simulink model "seti_ct"  (Simulink 6.2)
settings: Solver=ode45  StartTime=0.0  StopTime=100000  RelTol=1e-3
values from neighbouring files (symbols this model uses):
  bigColBits = 0    [address_gen_dram_mask.m]
  bigRowBits = log2(bigRowLength)    [address_gen_dram_mask.m]
  smallColBits = 0    [address_gen_dram_mask.m]
  smallRowBits = log2(smallRowLength)    [address_gen_dram_mask.m]
libraries: xbsIndex_r3 x487, xps_library x45, casper_library x18, fft_library x1
(part 1 of 3)
settings Model: LastModifiedBy=lspitler
settings DebuggingCC: SolverPrmCheckMsg=warning

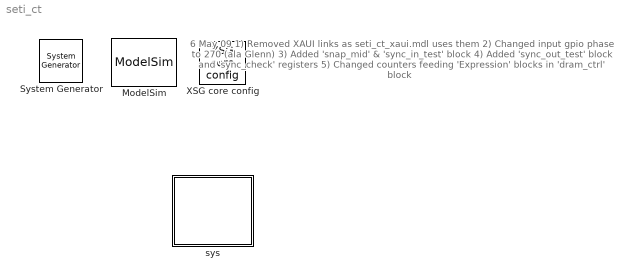
== system seti_ct ==
  note: 6 May 09
      | 1) Removed XAUI links as seti_ct_xaui.mdl uses them
      | 2) Changed input gpio phase to 270 (ala Glenn)
      | 3) Added 'snap_mid' & 'sync_in_test' block
      | 4) Added 'sync_out_test' block and 'sync_check' registers
      | 5) Changed counters feeding 'Expression' blocks
      | in 'dram_ctrl' block
  " System Generator" : xbsIndex_r3/ System Generator  Tag=genX  xilinxfamily=Virtex2P  part=xc2vp70  speed=-7  package=ff1704  synthesis_tool=XST  directory=./seti_ct/sysgen  testbench=off  simulink_period=1  sysclk_period=4.878  incr_netlist=off  trim_vbits=Everywhere in SubSystem  dbl_ovrd=According to Block Masks  core_generation=According to Block Masks  run_coregen=off  deprecated_control=off  eval_field=0
      settings: AttributesFormatString=System\nGenerator
  ModelSim : xbsIndex_r3/ModelSim  dir=./modelsim  waveform=on  leave_open=on  skip_compile=off  custom_scripts=on  post_vsim_script=dram_sim.do  startup_timeout=3600
  XSG core config : xps_library/XSG core config  Tag=xps:xsg  hw_sys=BEE2_usr  ibob_linux=off  clk_src=usr_clk2x  gpio_clk_io_group=iBOB:sma  gpio_clk_bit_index=0  clk_rate=205  sample_period=1  synthesis_tool=XST  mpc_type=powerpc405
  sys : Subsystem  mask{numSpecs=2^15, length=2^12, ct_delay=50}
      mask prompts: numSpecs "Number of Specs?"; length "Length of Specs?"; ct_delay "CornerTurn Delay"

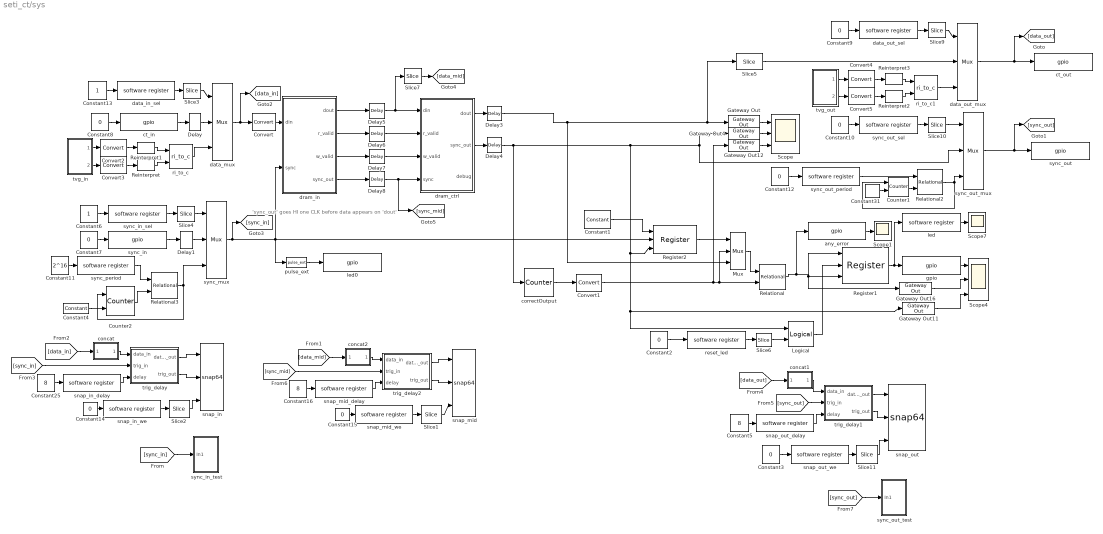
== system seti_ct/sys ==
  note: 'sync_out' goes HI
      | one CLK before
      | data appears on 'dout'
  Constant1 : xbsIndex_r3/Constant  const=1  equ=P=C  arith_type=Unsigned  n_bits=1  bin_pt=0  opselect=C  inp2=PCIN>>17  opr=+  inp1=P  carry=CIN  iostate=0  explicit_period=on  period=1  dbl_ovrd=off
  Constant{2..3,7..10,12,14..15} (9 alike) : Constant  Value=0
  Constant11 : Constant  Value=2^16
  Constant13 : Constant
  Constant16 : Constant  Value=8
  Constant25 : Constant  Value=8
  Constant31 : xbsIndex_r3/Constant  const=1  equ=P=C  arith_type=Unsigned  n_bits=32  bin_pt=0  opselect=C  inp2=PCIN>>17  opr=+  inp1=P  carry=CIN  iostate=0  explicit_period=on  period=1  dbl_ovrd=off
  Constant4 : xbsIndex_r3/Constant  const=1  equ=P=C  arith_type=Unsigned  n_bits=32  bin_pt=0  opselect=C  inp2=PCIN>>17  opr=+  inp1=P  carry=CIN  iostate=0  explicit_period=on  period=1  dbl_ovrd=off
  Constant5 : Constant  Value=8
  Constant6 : Constant
  Convert : xbsIndex_r3/Convert  arith_type=Unsigned  n_bits=72  bin_pt=0  quantization=Truncate  overflow=Wrap  latency=0  explicit_period=off  period=1  dbl_ovrd=off  show_param=off  inserted_by_tool=off  pipeline=off
      settings: xl_area=[0, 0, 0, 0, 0, 0, 0]
  Convert1 : xbsIndex_r3/Convert  arith_type=Unsigned  n_bits=72  bin_pt=0  quantization=Truncate  overflow=Wrap  latency=0  explicit_period=off  period=1  dbl_ovrd=off  show_param=off  inserted_by_tool=off  pipeline=off
      settings: xl_area=[0, 0, 0, 0, 0, 0, 0]
  Convert{2..5} (4 alike) : xbsIndex_r3/Convert  arith_type=Unsigned  n_bits=18  bin_pt=0  quantization=Truncate  overflow=Wrap  latency=0  explicit_period=on  period=1  dbl_ovrd=off  show_param=off  inserted_by_tool=off  pipeline=off
      settings: xl_area=[0, 0, 0, 0, 0, 0, 0]
  Counter1 : xbsIndex_r3/Counter  cnt_type=Free Running  n_bits=32  bin_pt=0  arith_type=Unsigned  start_count=0  cnt_to=Inf  cnt_by_val=1  operation=Up  explicit_period=on  period=1  load_pin=on  rst=off  en=off  dbl_ovrd=off  show_param=off  use_rpm=on  gen_core=off
      settings: xl_area=[0, 0, 0, 0, 0, 0, 0]
  Counter2 : xbsIndex_r3/Counter  cnt_type=Free Running  n_bits=32  bin_pt=0  arith_type=Unsigned  start_count=0  cnt_to=Inf  cnt_by_val=1  operation=Up  explicit_period=on  period=1  load_pin=on  rst=off  en=off  dbl_ovrd=off  show_param=off  use_rpm=on  gen_core=off
      settings: xl_area=[0, 0, 0, 0, 0, 0, 0]
  Delay{,1,3..8} (8 alike) : xbsIndex_r3/Delay  latency=1  reg_retiming=off  explicit_period=off  period=1  en=off  accept_only_valid=off  init_zero=on  dbl_ovrd=off  show_param=off
      settings: xl_area=[0, 0, 0, 0, 0, 0, 0]
  Gateway Out{,4,11..12,16} (5 alike) : xbsIndex_r3/Gateway Out  output_type=Double  nbits=8  bin_pt=6  arith_type=Boolean  quantization=Truncate  overflow=Wrap  hdl_port=off  timing_constraint=None  locs_specified=off  LOCs={}  needs_fixed_name=off  show_param=off
      settings: xl_area=[0, 0, 0, 0, 0, 0, 0]
  Logical : xbsIndex_r3/Logical  logical_function=AND  inputs=2  precision=Full  arith_type=Unsigned  n_bits=8  bin_pt=2  align_bp=on  latency=0  explicit_period=off  period=1  en=off  dbl_ovrd=off  show_param=off
      settings: xl_area=[0, 0, 0, 0, 0, 0, 0]
  Mux : xbsIndex_r3/Mux  inputs=2  precision=Full  arith_type="Signed  (2's comp)"  n_bits=8  bin_pt=2  quantization=Truncate  overflow=Wrap  latency=0  explicit_period=off  period=1  en=off  dbl_ovrd=off  show_param=off  mux_type=off  use_rpm=off  gen_core=off
      settings: xl_area=[0, 0, 0, 0, 0, 0, 0]
  Register1 : xbsIndex_r3/Register  init=0  reg_only_valid=off  explicit_period=off  period=1  rst=on  en=on  out_en=off  dbl_ovrd=off  show_param=off
      settings: xl_area=[0, 0, 0, 0, 0, 0, 0]
  Register2 : xbsIndex_r3/Register  init=0  reg_only_valid=off  explicit_period=off  period=1  rst=on  en=on  out_en=off  dbl_ovrd=off  show_param=off
      settings: xl_area=[0, 0, 0, 0, 0, 0, 0]
  Reinterpret{,1..3} (4 alike) : xbsIndex_r3/Reinterpret  force_arith_type=on  arith_type="Signed  (2's comp)"  force_bin_pt=on  bin_pt=17  force_valid=on
  Relational : xbsIndex_r3/Relational  mode=a!=b  latency=1  explicit_period=off  period=1  en=off  dbl_ovrd=off  show_param=off
      settings: xl_area=[0, 0, 0, 0, 0, 0, 0]
  Relational2 : xbsIndex_r3/Relational  mode=a=b  latency=1  explicit_period=off  period=1  en=off  dbl_ovrd=off  show_param=off
      settings: xl_area=[0, 0, 0, 0, 0, 0, 0]
  Relational3 : xbsIndex_r3/Relational  mode=a=b  latency=1  explicit_period=on  period=1  en=off  dbl_ovrd=off  show_param=off
      settings: xl_area=[0, 0, 0, 0, 0, 0, 0]
  Scope : Scope  NumInputPorts=3
      settings: YMin=-1~-1~0  YMax=1~1~1750  SaveName=ScopeData9
  Scope1 : Scope
      settings: SaveName=ScopeData12
  Scope4 : Scope  NumInputPorts=3
      settings: YMin=-1~-1~-1  YMax=1~1~1  SaveName=ScopeData10
  Scope7 : Scope
      settings: SaveName=ScopeData13
  Slice{1..2,6,11} (4 alike) : xbsIndex_r3/Slice  mode=Lower Bit Location + Width  nbits=1  bit1=0  base1=MSB of Input  bit0=0  base0=LSB of Input  boolean_output=on  explicit_period=off  period=1  dbl_ovrd=off
  Slice{3..4,9..10} (4 alike) : xbsIndex_r3/Slice  mode=Lower Bit Location + Width  nbits=1  bit1=0  base1=MSB of Input  bit0=0  base0=LSB of Input  boolean_output=off  explicit_period=off  period=1  dbl_ovrd=off
  Slice5 : xbsIndex_r3/Slice  mode=Lower Bit Location + Width  nbits=36  bit1=0  base1=MSB of Input  bit0=0  base0=LSB of Input  boolean_output=off  explicit_period=off  period=1  dbl_ovrd=off
  Slice7 : xbsIndex_r3/Slice  mode=Lower Bit Location + Width  nbits=36  bit1=0  base1=MSB of Input  bit0=0  base0=LSB of Input  boolean_output=off  explicit_period=off  period=1  dbl_ovrd=off
  any_error : xps_library/gpio  Tag=xps:gpio  io_group=BEE2_usr:led  io_dir=out  arith_type=Unsigned  bitwidth=1  bin_pt=0  bit_index=4  sample_period=1  use_single_ended=off  use_ddr=off  reg_iob=off  reg_clk_phase=0  termination=None
  concat : Subsystem
  concat1 : Subsystem
  concat2 : Subsystem
  correctOutput : xbsIndex_r3/Counter  cnt_type=Free Running  n_bits=log2(length)+log2(numSpecs)  bin_pt=0  arith_type=Unsigned  start_count=0  cnt_to=Inf  cnt_by_val=1  operation=Up  explicit_period=off  period=1  load_pin=off  rst=on  en=off  dbl_ovrd=off  show_param=off  use_rpm=on  gen_core=off
      settings: xl_area=[0, 0, 0, 0, 0, 0, 0]
  ct_in : xps_library/gpio  Tag=xps:gpio  io_group=BEE2_usr:rightlink  io_dir=in  arith_type=Unsigned  bitwidth=36  bin_pt=0  bit_index=[0:35]  sample_period=1  use_single_ended=off  use_ddr=off  reg_iob=on  reg_clk_phase=270  termination=None
  ct_out : xps_library/gpio  Tag=xps:gpio  io_group=BEE2_usr:leftlink  io_dir=out  arith_type=Unsigned  bitwidth=36  bin_pt=0  bit_index=[0:35]  sample_period=1  use_single_ended=off  use_ddr=off  reg_iob=on  reg_clk_phase=0  termination=None
  data_in_sel : xps_library/software register  Tag=xps:sw_reg  io_dir=From Processor  arith_type=Unsigned  bitwidth=32  bin_pt=0  sample_period=1  gw_name=seti_ct_sys_data_in_sel_user_data_out
  data_mux : xbsIndex_r3/Mux  inputs=2  precision=Full  arith_type="Signed  (2's comp)"  n_bits=8  bin_pt=2  quantization=Truncate  overflow=Wrap  latency=2  explicit_period=on  period=1  en=off  dbl_ovrd=off  show_param=off  mux_type=off  use_rpm=off  gen_core=off
      settings: xl_area=[0, 0, 0, 0, 0, 0, 0]
  data_out_mux : xbsIndex_r3/Mux  inputs=2  precision=Full  arith_type="Signed  (2's comp)"  n_bits=8  bin_pt=2  quantization=Truncate  overflow=Wrap  latency=2  explicit_period=on  period=1  en=off  dbl_ovrd=off  show_param=off  mux_type=off  use_rpm=off  gen_core=off
      settings: xl_area=[0, 0, 0, 0, 0, 0, 0]
  data_out_sel : xps_library/software register  Tag=xps:sw_reg  io_dir=From Processor  arith_type=Unsigned  bitwidth=32  bin_pt=0  sample_period=1  gw_name=seti_ct_sys_data_out_sel_user_data_out
  dram_ctrl : Subsystem  mask{spec_len=log2(length), num_spec=log2(numSpecs), ct_delay=ct_delay}
      mask prompts: spec_len "Spectrum Length (2^?)"; num_spec "Number of Spectra (2^?)"; ct_delay "Counterturn Delay"
  dram_in : Subsystem  mask{spec_len=log2(length)}
      mask prompts: spec_len "Spectrum Length (2^?)"
  gpio : xps_library/gpio  Tag=xps:gpio  io_group=BEE2_usr:led  io_dir=out  arith_type=Unsigned  bitwidth=1  bin_pt=0  bit_index=5  sample_period=1  use_single_ended=off  use_ddr=off  reg_iob=off  reg_clk_phase=0  termination=None
  led : xps_library/software register  Tag=xps:sw_reg  io_dir=To Processor  arith_type=Unsigned  bitwidth=32  bin_pt=0  sample_period=1  gw_name=seti_ct_sys_led_user_data_in
  led0 : xps_library/gpio  Tag=xps:gpio  io_group=BEE2_usr:led  io_dir=out  arith_type=Boolean  bitwidth=1  bin_pt=0  bit_index=0  sample_period=1  use_single_ended=off  use_ddr=off  reg_iob=on  reg_clk_phase=0  termination=None
  pulse_ext : casper_library/Misc/pulse_ext  pulse_len=2^25
  reset_led : xps_library/software register  Tag=xps:sw_reg  io_dir=From Processor  arith_type=Unsigned  bitwidth=32  bin_pt=0  sample_period=1  gw_name=seti_ct_sys_reset_led_user_data_out
  ri_to_c : casper_library/Misc/ri_to_c
  ri_to_c1 : casper_library/Misc/ri_to_c
  snap_in : casper_library/Scopes/snap64  nsamples=12
  snap_in_delay : xps_library/software register  Tag=xps:sw_reg  io_dir=From Processor  arith_type=Unsigned  bitwidth=32  bin_pt=0  sample_period=1  gw_name=seti_ct_sys_snap_in_delay_user_data_out
  snap_in_we : xps_library/software register  Tag=xps:sw_reg  io_dir=From Processor  arith_type=Unsigned  bitwidth=32  bin_pt=0  sample_period=1  gw_name=seti_ct_sys_snap_in_we_user_data_out
  snap_mid : casper_library/Scopes/snap64  nsamples=12
  snap_mid_delay : xps_library/software register  Tag=xps:sw_reg  io_dir=From Processor  arith_type=Unsigned  bitwidth=32  bin_pt=0  sample_period=1  gw_name=seti_ct_sys_snap_mid_delay_user_data_out
  snap_mid_we : xps_library/software register  Tag=xps:sw_reg  io_dir=From Processor  arith_type=Unsigned  bitwidth=32  bin_pt=0  sample_period=1  gw_name=seti_ct_sys_snap_mid_we_user_data_out
  snap_out : casper_library/Scopes/snap64  nsamples=11
  snap_out_delay : xps_library/software register  Tag=xps:sw_reg  io_dir=From Processor  arith_type=Unsigned  bitwidth=32  bin_pt=0  sample_period=1  gw_name=seti_ct_sys_snap_out_delay_user_data_out
  snap_out_we : xps_library/software register  Tag=xps:sw_reg  io_dir=From Processor  arith_type=Unsigned  bitwidth=32  bin_pt=0  sample_period=1  gw_name=seti_ct_sys_snap_out_we_user_data_out
  sync_in : xps_library/gpio  Tag=xps:gpio  io_group=BEE2_usr:rightlink  io_dir=in  arith_type=Boolean  bitwidth=1  bin_pt=0  bit_index=36  sample_period=1  use_single_ended=off  use_ddr=off  reg_iob=on  reg_clk_phase=270  termination=None
  sync_in_sel : xps_library/software register  Tag=xps:sw_reg  io_dir=From Processor  arith_type=Unsigned  bitwidth=32  bin_pt=0  sample_period=1  gw_name=seti_ct_sys_sync_in_sel_user_data_out
  sync_in_test : Subsystem
  sync_mux : xbsIndex_r3/Mux  inputs=2  precision=Full  arith_type="Signed  (2's comp)"  n_bits=8  bin_pt=2  quantization=Truncate  overflow=Wrap  latency=2  explicit_period=on  period=1  en=off  dbl_ovrd=off  show_param=off  mux_type=off  use_rpm=off  gen_core=off
      settings: xl_area=[0, 0, 0, 0, 0, 0, 0]
  sync_out : xps_library/gpio  Tag=xps:gpio  io_group=BEE2_usr:leftlink  io_dir=out  arith_type=Boolean  bitwidth=1  bin_pt=0  bit_index=36  sample_period=1  use_single_ended=off  use_ddr=off  reg_iob=on  reg_clk_phase=0  termination=None
  sync_out_mux : xbsIndex_r3/Mux  inputs=2  precision=Full  arith_type="Signed  (2's comp)"  n_bits=8  bin_pt=2  quantization=Truncate  overflow=Wrap  latency=2  explicit_period=on  period=1  en=off  dbl_ovrd=off  show_param=off  mux_type=off  use_rpm=off  gen_core=off
      settings: xl_area=[0, 0, 0, 0, 0, 0, 0]
  sync_out_period : xps_library/software register  Tag=xps:sw_reg  io_dir=From Processor  arith_type=Unsigned  bitwidth=32  bin_pt=0  sample_period=1  gw_name=seti_ct_sys_sync_out_period_user_data_out
  sync_out_sel : xps_library/software register  Tag=xps:sw_reg  io_dir=From Processor  arith_type=Unsigned  bitwidth=32  bin_pt=0  sample_period=1  gw_name=seti_ct_sys_sync_out_sel_user_data_out
  sync_out_test : Subsystem
  sync_period : xps_library/software register  Tag=xps:sw_reg  io_dir=From Processor  arith_type=Unsigned  bitwidth=32  bin_pt=0  sample_period=1  gw_name=seti_ct_sys_sync_period_user_data_out
  trig_delay : Subsystem
  trig_delay1 : Subsystem
  trig_delay2 : Subsystem
  tvg_in : Subsystem
  tvg_out : Subsystem
  wires:
  dram_in/2(r_valid) -> Delay6/1
  dram_in/3(w_valid) -> Delay7/1
  dram_in/4(sync_out) -> Delay8/1
  dram_in/1(dout) -> Delay5/1
  Convert/1 -> dram_in/1(din)
  dram_ctrl/1(dout) -> Delay3/1
  dram_ctrl/2(sync_out) -> Delay4/1
  Gateway Out/1 -> Scope/1
  correctOutput/1 -> Convert1/1
  Relational/1 -> Register1/3, Register1/1, Gateway Out16/1, any_error/1
  Register1/1 -> gpio/1, led/1
  gpio/1 -> Scope4/1
  Mux/1 -> Relational/1
  Register2/1 -> Mux/1
  Constant1/1 -> Register2/1
  Gateway Out12/1 -> Scope/3
  Gateway Out16/1 -> Scope4/2
  Gateway Out11/1 -> Scope4/3
  led/1 -> Scope7/1
  reset_led/1 -> Slice6/1
  Constant2/1 -> reset_led/1
  Slice6/1 -> Logical/2
  Logical/1 -> Register1/2
  any_error/1 -> Scope1/1
  Convert1/1 -> Relational/2, Mux/2, Gateway Out12/1
  data_in_sel/1 -> Slice3/1
  Constant13/1 -> data_in_sel/1
  Slice3/1 -> data_mux/1
  ri_to_c/1 -> data_mux/3
  ct_in/1 -> Delay/1
  sync_in_sel/1 -> Slice4/1
  Constant6/1 -> sync_in_sel/1
  Slice4/1 -> sync_mux/1
  sync_in/1 -> Delay1/1
  Constant7/1 -> sync_in/1
  sync_mux/1 -> Register2/2, dram_in/2(sync), pulse_ext/1, [sync_in]
  Constant8/1 -> ct_in/1
  Gateway Out4/1 -> Scope/2
  Convert2/1 -> Reinterpret1/1
  Convert3/1 -> Reinterpret/1
  tvg_in/1(re_out) -> Convert2/1
  tvg_in/2(im_out) -> Convert3/1
  Reinterpret1/1 -> ri_to_c/1
  Reinterpret/1 -> ri_to_c/2
  data_out_sel/1 -> Slice9/1
  Constant9/1 -> data_out_sel/1
  Slice9/1 -> data_out_mux/1
  ri_to_c1/1 -> data_out_mux/3
  Slice5/1 -> data_out_mux/2
  data_out_mux/1 -> [data_out], ct_out/1
  Convert4/1 -> Reinterpret3/1
  Convert5/1 -> Reinterpret2/1
  tvg_out/1(re_out) -> Convert4/1
  tvg_out/2(im_out) -> Convert5/1
  Reinterpret3/1 -> ri_to_c1/1
  Reinterpret2/1 -> ri_to_c1/2
  Relational2/1 -> Counter1/1, sync_out_mux/3
  sync_out_period/1 -> Relational2/1
  Counter1/1 -> Relational2/2
  sync_out_mux/1 -> [sync_out], sync_out/1
  sync_out_sel/1 -> Slice10/1
  Constant10/1 -> sync_out_sel/1
  Slice10/1 -> sync_out_mux/1
  Constant12/1 -> sync_out_period/1
  snap_out_we/1 -> Slice11/1
  Slice11/1 -> snap_out/3
  Constant3/1 -> snap_out_we/1
  Counter2/1 -> Relational3/2
  sync_period/1 -> Relational3/1
  Constant11/1 -> sync_period/1
  Constant4/1 -> Counter2/2
  Relational3/1 -> sync_mux/3, Counter2/1
  snap_in_we/1 -> Slice2/1
  Slice2/1 -> snap_in/3
  Constant14/1 -> snap_in_we/1
  pulse_ext/1 -> led0/1
  Constant25/1 -> snap_in_delay/1
  snap_in_delay/1 -> trig_delay/3(delay)
  concat/1(Out1) -> trig_delay/1(data_in)
  trig_delay/1(data_out) -> snap_in/1
  trig_delay/2(trig_out) -> snap_in/2
  [data_in] -> concat/1(In1)
  [sync_in] -> trig_delay/2(trig_in)
  Constant5/1 -> snap_out_delay/1
  snap_out_delay/1 -> trig_delay1/3(delay)
  concat1/1(Out1) -> trig_delay1/1(data_in)
  [data_out] -> concat1/1(In1)
  [sync_out] -> trig_delay1/2(trig_in)
  trig_delay1/1(data_out) -> snap_out/1
  trig_delay1/2(trig_out) -> snap_out/2
  Delay/1 -> data_mux/2
  Delay1/1 -> sync_mux/2
  Constant31/1 -> Counter1/2
  Delay3/1 -> Mux/3, Gateway Out/1, Slice5/1
  Delay4/1 -> Register2/3, Gateway Out11/1, Logical/1, Gateway Out4/1, sync_out_mux/2, correctOutput/1
  Delay5/1 -> dram_ctrl/1(din), Slice7/1
  Delay6/1 -> dram_ctrl/2(r_valid)
  Delay7/1 -> dram_ctrl/3(w_valid)
  Delay8/1 -> dram_ctrl/4(sync), [sync_mid]
  data_mux/1 -> Convert/1, [data_in]
  [sync_in] -> sync_in_test/1(In1)
  snap_mid_we/1 -> Slice1/1
  Slice1/1 -> snap_mid/3
  Constant15/1 -> snap_mid_we/1
  Constant16/1 -> snap_mid_delay/1
  snap_mid_delay/1 -> trig_delay2/3(delay)
  concat2/1(Out1) -> trig_delay2/1(data_in)
  trig_delay2/1(data_out) -> snap_mid/1
  trig_delay2/2(trig_out) -> snap_mid/2
  [data_mid] -> concat2/1(In1)
  [sync_mid] -> trig_delay2/2(trig_in)
  Slice7/1 -> [data_mid]
  [sync_out] -> sync_out_test/1(In1)

== system seti_ct/sys/concat ==
  In1 : Inport  Port=1  LatchInput=off
  Concat1 : xbsIndex_r3/Concat  num_inputs=4  explicit_period=on  period=1  dbl_ovrd=off
  Constant5 : xbsIndex_r3/Constant  const=0  equ=P=C  arith_type=Unsigned  n_bits=14  bin_pt=0  opselect=C  inp2=PCIN>>17  opr=+  inp1=P  carry=CIN  iostate=0  explicit_period=on  period=1  dbl_ovrd=off
  Slice7 : xbsIndex_r3/Slice  mode=Upper Bit Location + Width  nbits=18  bit1=0  base1=MSB of Input  bit0=0  base0=LSB of Input  boolean_output=off  explicit_period=off  period=1  dbl_ovrd=off
  Slice8 : xbsIndex_r3/Slice  mode=Lower Bit Location + Width  nbits=18  bit1=0  base1=MSB of Input  bit0=0  base0=LSB of Input  boolean_output=off  explicit_period=off  period=1  dbl_ovrd=off
  Out1 : Outport
  wires:
  Slice8/1 -> Concat1/4
  Slice7/1 -> Concat1/2
  Constant5/1 -> Concat1/1, Concat1/3
  Concat1/1 -> Out1/1
  In1/1 -> Slice7/1, Slice8/1

== system seti_ct/sys/concat1 ==
  In1 : Inport  Port=1  LatchInput=off
  Concat1 : xbsIndex_r3/Concat  num_inputs=4  explicit_period=on  period=1  dbl_ovrd=off
  Constant5 : xbsIndex_r3/Constant  const=0  equ=P=C  arith_type=Unsigned  n_bits=14  bin_pt=0  opselect=C  inp2=PCIN>>17  opr=+  inp1=P  carry=CIN  iostate=0  explicit_period=on  period=1  dbl_ovrd=off
  Slice7 : xbsIndex_r3/Slice  mode=Upper Bit Location + Width  nbits=18  bit1=0  base1=MSB of Input  bit0=0  base0=LSB of Input  boolean_output=off  explicit_period=off  period=1  dbl_ovrd=off
  Slice8 : xbsIndex_r3/Slice  mode=Lower Bit Location + Width  nbits=18  bit1=0  base1=MSB of Input  bit0=0  base0=LSB of Input  boolean_output=off  explicit_period=off  period=1  dbl_ovrd=off
  Out1 : Outport
  wires:
  Slice8/1 -> Concat1/4
  Slice7/1 -> Concat1/2
  Constant5/1 -> Concat1/1, Concat1/3
  Concat1/1 -> Out1/1
  In1/1 -> Slice7/1, Slice8/1

== system seti_ct/sys/concat2 ==
  In1 : Inport  Port=1  LatchInput=off
  Concat1 : xbsIndex_r3/Concat  num_inputs=4  explicit_period=on  period=1  dbl_ovrd=off
  Constant5 : xbsIndex_r3/Constant  const=0  equ=P=C  arith_type=Unsigned  n_bits=14  bin_pt=0  opselect=C  inp2=PCIN>>17  opr=+  inp1=P  carry=CIN  iostate=0  explicit_period=on  period=1  dbl_ovrd=off
  Slice7 : xbsIndex_r3/Slice  mode=Upper Bit Location + Width  nbits=18  bit1=0  base1=MSB of Input  bit0=0  base0=LSB of Input  boolean_output=off  explicit_period=off  period=1  dbl_ovrd=off
  Slice8 : xbsIndex_r3/Slice  mode=Lower Bit Location + Width  nbits=18  bit1=0  base1=MSB of Input  bit0=0  base0=LSB of Input  boolean_output=off  explicit_period=off  period=1  dbl_ovrd=off
  Out1 : Outport
  wires:
  Slice8/1 -> Concat1/4
  Slice7/1 -> Concat1/2
  Constant5/1 -> Concat1/1, Concat1/3
  Concat1/1 -> Out1/1
  In1/1 -> Slice7/1, Slice8/1

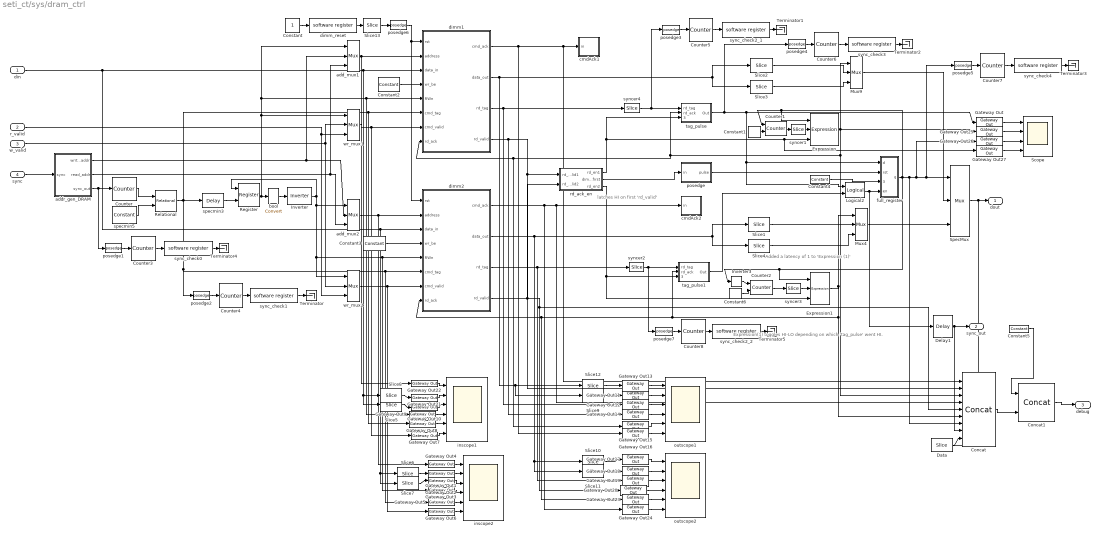
== system seti_ct/sys/dram_ctrl ==
  note: Added a latency
      | of 1 to 'Expression (1)'
  note: latches HI on
      | first 'rd_valid'
  note: Expression(1) toggles
      | HI-LO depending
      | on which 'tag_pulse'
      | went HI.
  din : Inport  Port=1  LatchInput=off
  r_valid : Inport  Port=2  LatchInput=off
  w_valid : Inport  Port=3  LatchInput=off
  sync : Inport  Port=4  LatchInput=off
  Concat : xbsIndex_r3/Concat  num_inputs=9  explicit_period=off  period=1  dbl_ovrd=off
  Concat1 : xbsIndex_r3/Concat  num_inputs=2  explicit_period=off  period=1  dbl_ovrd=off
  Constant : Constant
  Constant1 : xbsIndex_r3/Constant  const=1  equ=P=C  arith_type=Unsigned  n_bits=2  bin_pt=0  opselect=C  inp2=PCIN>>17  opr=+  inp1=P  carry=CIN  iostate=0  explicit_period=on  period=1  dbl_ovrd=off
  Constant2 : xbsIndex_r3/Constant  const=2^18-1  equ=P=C  arith_type=Unsigned  n_bits=18  bin_pt=0  opselect=C  inp2=PCIN>>17  opr=+  inp1=P  carry=CIN  iostate=0  explicit_period=on  period=1  dbl_ovrd=off
  Constant3 : xbsIndex_r3/Constant  const=2^18-1  equ=P=C  arith_type=Unsigned  n_bits=18  bin_pt=0  opselect=C  inp2=PCIN>>17  opr=+  inp1=P  carry=CIN  iostate=0  explicit_period=on  period=1  dbl_ovrd=off
  Constant4 : xbsIndex_r3/Constant  const=0  equ=P=C  arith_type=Boolean  n_bits=1  bin_pt=0  opselect=C  inp2=PCIN>>17  opr=+  inp1=P  carry=CIN  iostate=0  explicit_period=off  period=1  dbl_ovrd=off
  Constant5 : xbsIndex_r3/Constant  const=0  equ=P=C  arith_type=Unsigned  n_bits=8  bin_pt=0  opselect=C  inp2=PCIN>>17  opr=+  inp1=P  carry=CIN  iostate=0  explicit_period=off  period=1  dbl_ovrd=off
  Constant6 : xbsIndex_r3/Constant  const=1  equ=P=C  arith_type=Unsigned  n_bits=2  bin_pt=0  opselect=C  inp2=PCIN>>17  opr=+  inp1=P  carry=CIN  iostate=0  explicit_period=on  period=1  dbl_ovrd=off
  Counter : xbsIndex_r3/Counter  cnt_type=Free Running  n_bits=spec_len + num_spec  bin_pt=0  arith_type=Unsigned  start_count=0  cnt_to=Inf  cnt_by_val=1  operation=Up  explicit_period=off  period=1  load_pin=off  rst=on  en=off  dbl_ovrd=off  show_param=off  use_rpm=on  gen_core=off
      settings: xl_area=[0, 0, 0, 0, 0, 0, 0]
  Counter1 : xbsIndex_r3/Counter  cnt_type=Free Running  n_bits=2  bin_pt=0  arith_type=Unsigned  start_count=0  cnt_to=Inf  cnt_by_val=1  operation=Up  explicit_period=off  period=1  load_pin=on  rst=off  en=off  dbl_ovrd=off  show_param=off  use_rpm=on  gen_core=off
      settings: xl_area=[0, 0, 0, 0, 0, 0, 0]
  Counter2 : xbsIndex_r3/Counter  cnt_type=Free Running  n_bits=2  bin_pt=0  arith_type=Unsigned  start_count=0  cnt_to=Inf  cnt_by_val=1  operation=Up  explicit_period=off  period=1  load_pin=on  rst=off  en=off  dbl_ovrd=off  show_param=off  use_rpm=on  gen_core=off
      settings: xl_area=[0, 0, 0, 0, 0, 0, 0]
  Counter{3..8} (6 alike) : xbsIndex_r3/Counter  cnt_type=Free Running  n_bits=32  bin_pt=0  arith_type=Unsigned  start_count=0  cnt_to=Inf  cnt_by_val=1  operation=Up  explicit_period=on  period=1  load_pin=off  rst=off  en=on  dbl_ovrd=off  show_param=off  use_rpm=on  gen_core=off
      settings: xl_area=[0, 0, 0, 0, 0, 0, 0]
  Data : xbsIndex_r3/Slice  mode=Lower Bit Location + Width  nbits=16  bit1=0  base1=MSB of Input  bit0=0  base0=LSB of Input  boolean_output=off  explicit_period=off  period=1  dbl_ovrd=off
  Delay1 : xbsIndex_r3/Delay  latency=1  reg_retiming=off  explicit_period=off  period=1  en=off  accept_only_valid=off  init_zero=on  dbl_ovrd=off  show_param=off
      settings: xl_area=[0, 0, 0, 0, 0, 0, 0]
  Expression : xbsIndex_r3/Expression  expression=~a & b & c  precision=Full  arith_type=Unsigned  n_bits=8  bin_pt=2  align_bp=on  latency=1  explicit_period=off  period=1  en=off  dbl_ovrd=off  show_param=off
      settings: xl_area=[0, 0, 0, 0, 0, 0, 0]
  Expression1 : xbsIndex_r3/Expression  expression=a & b & c  precision=Full  arith_type=Unsigned  n_bits=8  bin_pt=2  align_bp=on  latency=1  explicit_period=off  period=1  en=off  dbl_ovrd=off  show_param=off
      settings: xl_area=[0, 0, 0, 0, 0, 0, 0]
  Gateway Out{,25..27} (4 alike) : xbsIndex_r3/Gateway Out  output_type=Double  nbits=8  bin_pt=6  arith_type=Boolean  quantization=Truncate  overflow=Wrap  hdl_port=on  timing_constraint=None  locs_specified=off  LOCs={}  needs_fixed_name=off  show_param=off
      settings: xl_area=[0, 0, 0, 0, 0, 0, 0]
  Gateway Out{1..24} (24 alike) : xbsIndex_r3/Gateway Out  output_type=Double  nbits=8  bin_pt=6  arith_type=Boolean  quantization=Truncate  overflow=Wrap  hdl_port=off  timing_constraint=None  locs_specified=off  LOCs={}  needs_fixed_name=off  show_param=off
      settings: xl_area=[0, 0, 0, 0, 0, 0, 0]
  Inverter : xbsIndex_r3/Inverter  latency=0  explicit_period=off  period=1  en=off  dbl_ovrd=off  show_param=off
      settings: xl_area=[0, 0, 0, 0, 0, 0, 0]
  Inverter3 : xbsIndex_r3/Inverter  latency=0  explicit_period=off  period=1  en=off  dbl_ovrd=off  show_param=off
      settings: xl_area=[0, 0, 0, 0, 0, 0, 0]
  Logical2 : xbsIndex_r3/Logical  logical_function=OR  inputs=2  precision=Full  arith_type=Unsigned  n_bits=8  bin_pt=2  align_bp=on  latency=0  explicit_period=off  period=1  en=off  dbl_ovrd=off  show_param=off
      settings: xl_area=[0, 0, 0, 0, 0, 0, 0]
  Mux4 : xbsIndex_r3/Mux  inputs=2  precision=Full  arith_type="Signed  (2's comp)"  n_bits=8  bin_pt=2  quantization=Truncate  overflow=Wrap  latency=0  explicit_period=off  period=1  en=off  dbl_ovrd=off  show_param=off  mux_type=off  use_rpm=off  gen_core=off
      settings: xl_area=[0, 0, 0, 0, 0, 0, 0]
  Mux9 : xbsIndex_r3/Mux  inputs=2  precision=Full  arith_type="Signed  (2's comp)"  n_bits=8  bin_pt=2  quantization=Truncate  overflow=Wrap  latency=0  explicit_period=off  period=1  en=off  dbl_ovrd=off  show_param=off  mux_type=off  use_rpm=off  gen_core=off
      settings: xl_area=[0, 0, 0, 0, 0, 0, 0]
  Register : xbsIndex_r3/Register  init=0  reg_only_valid=off  explicit_period=off  period=1  rst=off  en=on  out_en=off  dbl_ovrd=off  show_param=off
      settings: xl_area=[0, 0, 0, 0, 0, 0, 0]
  Relational : xbsIndex_r3/Relational  mode=a=b  latency=1  explicit_period=off  period=1  en=off  dbl_ovrd=off  show_param=off
      settings: xl_area=[0, 0, 0, 0, 0, 0, 0]
  Scope : Scope  NumInputPorts=4
      settings: YMin=-5~-5~-5~-5  YMax=5~5~5~5  SaveName=ScopeData11
  Slice{1..2,5,7,9,11} (6 alike) : xbsIndex_r3/Slice  mode=Lower Bit Location + Width  nbits=72  bit1=0  base1=MSB of Input  bit0=0  base0=LSB of Input  boolean_output=off  explicit_period=off  period=1  dbl_ovrd=off
  Slice{3..4,6,8,10,12} (6 alike) : xbsIndex_r3/Slice  mode=Upper Bit Location + Width  nbits=72  bit1=0  base1=MSB of Input  bit0=0  base0=LSB of Input  boolean_output=off  explicit_period=off  period=1  dbl_ovrd=off
  Slice13 : xbsIndex_r3/Slice  mode=Lower Bit Location + Width  nbits=1  bit1=0  base1=MSB of Input  bit0=0  base0=LSB of Input  boolean_output=on  explicit_period=off  period=1  dbl_ovrd=off
  SpecMux : xbsIndex_r3/Mux  inputs=2  precision=Full  arith_type="Signed  (2's comp)"  n_bits=8  bin_pt=2  quantization=Truncate  overflow=Wrap  latency=1  explicit_period=off  period=1  en=off  dbl_ovrd=off  show_param=off  mux_type=off  use_rpm=off  gen_core=off
      settings: xl_area=[0, 0, 0, 0, 0, 0, 0]
  Terminator{,1..5} (6 alike) : Terminator
  add_mux1 : xbsIndex_r3/Mux  inputs=2  precision=Full  arith_type="Signed  (2's comp)"  n_bits=8  bin_pt=2  quantization=Truncate  overflow=Wrap  latency=0  explicit_period=off  period=1  en=off  dbl_ovrd=off  show_param=off  mux_type=off  use_rpm=off  gen_core=off
      settings: xl_area=[0, 0, 0, 0, 0, 0, 0]
  add_mux2 : xbsIndex_r3/Mux  inputs=2  precision=Full  arith_type="Signed  (2's comp)"  n_bits=8  bin_pt=2  quantization=Truncate  overflow=Wrap  latency=0  explicit_period=off  period=1  en=off  dbl_ovrd=off  show_param=off  mux_type=off  use_rpm=off  gen_core=off
      settings: xl_area=[0, 0, 0, 0, 0, 0, 0]
  addr_gen_DRAM : Subsystem  mask{numSpecs=2^num_spec, length=2^spec_len}
      mask prompts: numSpecs "Number of Spectrums?"; length "Length of Spectrum?"
      mask init:
      | address_gen_dram_mask;
  bool : xbsIndex_r3/Convert  arith_type=Boolean  n_bits=8  bin_pt=6  quantization=Truncate  overflow=Wrap  latency=0  explicit_period=on  period=1  dbl_ovrd=off  show_param=off  inserted_by_tool=off  pipeline=off
      settings: xl_area=[0, 0, 0, 0, 0, 0, 0]
  cmdAck1 : Subsystem
  cmdAck2 : Subsystem
  dimm1 : Subsystem  Tag=xps:dram  AncestorBlock=xps_library/dram  mask(dram){dimm=1, arith_type=Unsigned, bin_pt=0, ip_clock=200, sample_period=1, use_sim=on, bank_mgt=off, wide_data=off, half_burst=off}
      mask prompts: arith_type "Data Type"; bin_pt "Data binary point"; ip_clock "Datapath clock rate (MHz)"; sample_period "Sample period"; use_sim "Simulate DRAM using ModelSim"; bank_mgt "Enable bank management"; wide_data "Use wide data bus (288 bits)"; half_burst "Use half-burst"
      mask help:
      | Interface to 1GB DDR2 DIMMs on BEE2.
      |
      | To simulate using ModelSim, place a ModelSim block named 'ModelSim' (case-sensitive) in the top level of the design.
      mask init:
      | dram_mask;
      mask StyleString: popup(1|2|3|4),popup(Boolean|Unsigned|Signed  (2's comp)),edit,edit,edit,checkbox,checkbox,checkbox,checkbox
      mask CallbackString:
      | |||||||myname=gcb;
      | if strcmp(get_param(myname, 'wide_data'), 'off')
      |     set_param(myname, 'MaskEnables', {'on','on','on','on','on','on','on','on','on'});
      | else
      |     set_param(myname, 'half_burst', 'off');
      |     set_param(myname, 'MaskEnables', {'on','on','on','on','on','on','on','on','off'});
      | end|
  dimm2 : Subsystem  Tag=xps:dram  AncestorBlock=xps_library/dram  mask(dram){dimm=2, arith_type=Unsigned, bin_pt=0, ip_clock=200, sample_period=1, use_sim=on, bank_mgt=off, wide_data=off, half_burst=off}
      mask prompts: arith_type "Data Type"; bin_pt "Data binary point"; ip_clock "Datapath clock rate (MHz)"; sample_period "Sample period"; use_sim "Simulate DRAM using ModelSim"; bank_mgt "Enable bank management"; wide_data "Use wide data bus (288 bits)"; half_burst "Use half-burst"
      mask help:
      | Interface to 1GB DDR2 DIMMs on BEE2.
      |
      | To simulate using ModelSim, place a ModelSim block named 'ModelSim' (case-sensitive) in the top level of the design.
      mask init:
      | dram_mask;
      mask StyleString: popup(1|2|3|4),popup(Boolean|Unsigned|Signed  (2's comp)),edit,edit,edit,checkbox,checkbox,checkbox,checkbox
      mask CallbackString:
      | |||||||myname=gcb;
      | if strcmp(get_param(myname, 'wide_data'), 'off')
      |     set_param(myname, 'MaskEnables', {'on','on','on','on','on','on','on','on','on'});
      | else
      |     set_param(myname, 'half_burst', 'off');
      |     set_param(myname, 'MaskEnables', {'on','on','on','on','on','on','on','on','off'});
      | end|
  dimm_reset : xps_library/software register  Tag=xps:sw_reg  io_dir=From Processor  arith_type=Unsigned  bitwidth=32  bin_pt=0  sample_period=1  gw_name=seti_ct_sys_dram_ctrl_dimm_reset_user_data_out
  full_register : Subsystem  mask{num_bits=1, init_val=1}
      mask prompts: num_bits "Number of Bits"; init_val "Initial Value"
  inscope1 : Scope  NumInputPorts=6
      settings: TimeRange=45.11589403973511  YMin=0~0~0~0~0~-5  YMax=157.8428582181891~4.1454e+022~1~1~1~5  SaveName=ScopeData4
  inscope2 : Scope  NumInputPorts=6
      settings: TimeRange=45.11589403973511  YMin=0~0~0~0~0~-5  YMax=157.8428582181891~4.1454e+022~1~1~1~5  SaveName=ScopeData5
  outscope1 : Scope  NumInputPorts=6
      settings: TimeRange=45.11589403973511  YMin=1295~1295~-1~0.95~0~0  YMax=1335~1335~1~1.05~1~1  SaveName=ScopeData6
  outscope2 : Scope  NumInputPorts=6
      settings: TimeRange=45.11589403973511  YMin=-1~-1~-1~0~0~0  YMax=1~1~1~1~1~1  SaveName=ScopeData3
  posedge : Subsystem
  posedge{1..7} (7 alike) : casper_library/Misc/posedge  Tag=Rising Edge Detector
  rd_ack_en : Subsystem  mask{ct_delay=ct_delay}
      mask prompts: ct_delay "Corner Turn Delay"
  specmin3 : xbsIndex_r3/Delay  latency=2  reg_retiming=off  explicit_period=off  period=1  en=off  accept_only_valid=off  init_zero=on  dbl_ovrd=off  show_param=off
      settings: xl_area=[0, 0, 0, 0, 0, 0, 0]
  specmin5 : xbsIndex_r3/Constant  const=2^(spec_len+num_spec) -5  equ=P=C  arith_type=Unsigned  n_bits=(spec_len+num_spec)  bin_pt=0  opselect=C  inp2=PCIN>>17  opr=+  inp1=P  carry=CIN  iostate=0  explicit_period=off  period=1  dbl_ovrd=off
  sync_check0 : xps_library/software register  Tag=xps:sw_reg  io_dir=To Processor  arith_type=Unsigned  bitwidth=32  bin_pt=0  sample_period=1  gw_name=seti_ct_sys_dram_ctrl_sync_check0_user_data_in
  sync_check1 : xps_library/software register  Tag=xps:sw_reg  io_dir=To Processor  arith_type=Unsigned  bitwidth=32  bin_pt=0  sample_period=1  gw_name=seti_ct_sys_dram_ctrl_sync_check1_user_data_in
  sync_check2_1 : xps_library/software register  Tag=xps:sw_reg  io_dir=To Processor  arith_type=Unsigned  bitwidth=32  bin_pt=0  sample_period=1  gw_name=seti_ct_sys_dram_ctrl_sync_check2_1_user_data_in
  sync_check2_2 : xps_library/software register  Tag=xps:sw_reg  io_dir=To Processor  arith_type=Unsigned  bitwidth=32  bin_pt=0  sample_period=1  gw_name=seti_ct_sys_dram_ctrl_sync_check2_2_user_data_in
  sync_check3 : xps_library/software register  Tag=xps:sw_reg  io_dir=To Processor  arith_type=Unsigned  bitwidth=32  bin_pt=0  sample_period=1  gw_name=seti_ct_sys_dram_ctrl_sync_check3_user_data_in
  sync_check4 : xps_library/software register  Tag=xps:sw_reg  io_dir=To Processor  arith_type=Unsigned  bitwidth=32  bin_pt=0  sample_period=1  gw_name=seti_ct_sys_dram_ctrl_sync_check4_user_data_in
  syncer{1..4} (4 alike) : xbsIndex_r3/Slice  mode=Lower Bit Location + Width  nbits=1  bit1=0  base1=MSB of Input  bit0=0  base0=LSB of Input  boolean_output=on  explicit_period=on  period=1  dbl_ovrd=off
  tag_pulse : Subsystem
  tag_pulse1 : Subsystem
  wr_mux1 : xbsIndex_r3/Mux  inputs=2  precision=Full  arith_type="Signed  (2's comp)"  n_bits=8  bin_pt=2  quantization=Truncate  overflow=Wrap  latency=0  explicit_period=off  period=1  en=off  dbl_ovrd=off  show_param=off  mux_type=off  use_rpm=off  gen_core=off
      settings: xl_area=[0, 0, 0, 0, 0, 0, 0]
  wr_mux2 : xbsIndex_r3/Mux  inputs=2  precision=Full  arith_type="Signed  (2's comp)"  n_bits=8  bin_pt=2  quantization=Truncate  overflow=Wrap  latency=0  explicit_period=off  period=1  en=off  dbl_ovrd=off  show_param=off  mux_type=off  use_rpm=off  gen_core=off
      settings: xl_area=[0, 0, 0, 0, 0, 0, 0]
  dout : Outport
  sync_out : Outport  Port=2
  debug : Outport  Port=3
  wires:
  addr_gen_DRAM/2(read_addr) -> add_mux1/3, add_mux2/3
  add_mux1/1 -> dimm1/2(address), Gateway Out22/1
  add_mux2/1 -> dimm2/2(address), Gateway Out4/1
  Constant2/1 -> dimm1/4(wr_be)
  Constant3/1 -> dimm2/4(wr_be)
  addr_gen_DRAM/3(sync_out) -> Counter/1, posedge1/1
  Register/1 -> add_mux1/1, dimm1/5(RWn), Gateway Out9/1, wr_mux1/1, bool/1
  Inverter/1 -> add_mux2/1, wr_mux2/1, dimm2/5(RWn), Gateway Out3/1, Register/1
  Counter/1 -> Relational/1
  specmin5/1 -> Relational/2
  Relational/1 -> dimm1/6(cmd_tag), Gateway Out8/1, specmin3/1, dimm2/6(cmd_tag), Gateway Out5/1, posedge2/1
  din/1 -> dimm1/3(data_in), Slice8/1, Slice5/1, dimm2/3(data_in), Slice6/1, Slice7/1
  sync/1 -> addr_gen_DRAM/1(sync)
  r_valid/1 -> wr_mux2/3, wr_mux1/3
  wr_mux1/1 -> dimm1/7(cmd_valid), Gateway Out7/1
  wr_mux2/1 -> dimm2/7(cmd_valid), Gateway Out6/1
  w_valid/1 -> wr_mux2/2, wr_mux1/2
  dimm1/3(rd_tag) -> syncer4/1, Gateway Out12/1
  dimm2/3(rd_tag) -> syncer2/1, Gateway Out19/1
  bool/1 -> Inverter/1
  Gateway Out22/1 -> inscope1/1
  Gateway Out21/1 -> inscope1/2
  Gateway Out10/1 -> inscope1/3
  Gateway Out9/1 -> inscope1/4
  Gateway Out8/1 -> inscope1/5
  Gateway Out4/1 -> inscope2/1
  Gateway Out1/1 -> inscope2/2
  Gateway Out2/1 -> inscope2/3
  Gateway Out3/1 -> inscope2/4
  Gateway Out5/1 -> inscope2/5
  Slice5/1 -> Gateway Out10/1
  Slice6/1 -> Gateway Out1/1
  Slice7/1 -> Gateway Out2/1
  Slice9/1 -> Gateway Out11/1
  Gateway Out12/1 -> outscope1/3
  Gateway Out14/1 -> outscope1/4
  Gateway Out15/1 -> outscope1/5
  Slice10/1 -> Gateway Out17/1
  Slice11/1 -> Gateway Out18/1
  Gateway Out13/1 -> outscope1/1
  Gateway Out11/1 -> outscope1/2
  dimm1/1(cmd_ack) -> Gateway Out16/1, cmdAck1/1(in), Concat/1
  dimm2/1(cmd_ack) -> Gateway Out24/1, cmdAck2/1(in), Concat/4
  dimm2/4(rd_valid) -> rd_ack_en/2(rd_valid2), Gateway Out20/1, Concat/5
  dimm1/4(rd_valid) -> Gateway Out14/1, rd_ack_en/1(rd_valid1), Concat/2
  dimm1/2(data_out) -> Slice12/1, Slice9/1, Slice2/1, Slice3/1
  dimm2/2(data_out) -> Slice10/1, Slice11/1, Slice4/1, Slice1/1
  Slice8/1 -> Gateway Out21/1
  Slice12/1 -> Gateway Out13/1
  Gateway Out7/1 -> inscope1/6
  Gateway Out16/1 -> outscope1/6
  Gateway Out19/1 -> outscope2/3
  Gateway Out20/1 -> outscope2/4
  Gateway Out23/1 -> outscope2/5
  Gateway Out17/1 -> outscope2/1
  Gateway Out18/1 -> outscope2/2
  Slice2/1 -> Mux9/2
  Slice3/1 -> Mux9/3
  Slice1/1 -> Mux4/2
  Slice4/1 -> Mux4/3
  Gateway Out6/1 -> inscope2/6
  Gateway Out24/1 -> outscope2/6
  Logical2/1 -> Delay1/1, full_register/4(en)
  tag_pulse1/1(Out) -> Logical2/2
  full_register/1(q) -> Inverter3/1, Expression1/1, Counter1/1, Expression/1, Gateway Out26/1, SpecMux/1, posedge5/1, Concat/7
  Mux9/1 -> SpecMux/2
  Mux4/1 -> SpecMux/3
  SpecMux/1 -> dout/1, Data/1
  Inverter3/1 -> Counter2/1
  Expression/1 -> Mux9/1, dimm1/8(rd_ack), Gateway Out15/1, tag_pulse/2(rd_ack), Concat/3, Gateway Out25/1
  Expression1/1 -> Mux4/1, dimm2/8(rd_ack), Gateway Out23/1, tag_pulse1/2(rd_ack), Concat/6
  Counter1/1 -> syncer1/1
  Counter2/1 -> syncer3/1
  syncer1/1 -> Expression/2
  syncer3/1 -> Expression1/2
  addr_gen_DRAM/1(write_addr) -> add_mux2/2, add_mux1/2
  syncer4/1 -> tag_pulse/1(rd_tag), posedge3/1
  syncer2/1 -> tag_pulse1/1(rd_tag), posedge7/1
  Delay1/1 -> sync_out/1, Concat/8
  rd_ack_en/1(rd_en1) -> tag_pulse/3(rd_valid), Expression/3, Gateway Out27/1
  rd_ack_en/3(rd_en2) -> tag_pulse1/3(rd_valid), Expression1/3
  rd_ack_en/2(dimm1_first) -> posedge/1(in)
  tag_pulse/1(Out) -> posedge4/1, Logical2/1, full_register/1(d), Gateway Out/1
  posedge/1(pulse) -> full_register/2(rst)
  Constant4/1 -> full_register/3(set)
  specmin3/1 -> Register/2
  Data/1 -> Concat/9
  Concat/1 -> Concat1/2
  Concat1/1 -> debug/1
  Constant5/1 -> Concat1/1
  Gateway Out/1 -> Scope/1
  Gateway Out25/1 -> Scope/2
  Gateway Out26/1 -> Scope/3
  Gateway Out27/1 -> Scope/4
  dimm_reset/1 -> Slice13/1
  Constant/1 -> dimm_reset/1
  Counter3/1 -> sync_check0/1
  posedge1/1 -> Counter3/1
  Counter4/1 -> sync_check1/1
  posedge2/1 -> Counter4/1
  Counter5/1 -> sync_check2_1/1
  posedge3/1 -> Counter5/1
  Counter6/1 -> sync_check3/1
  posedge4/1 -> Counter6/1
  Counter7/1 -> sync_check4/1
  posedge5/1 -> Counter7/1
  sync_check1/1 -> Terminator/1
  sync_check2_1/1 -> Terminator1/1
  sync_check3/1 -> Terminator2/1
  sync_check4/1 -> Terminator3/1
  sync_check0/1 -> Terminator4/1
  Slice13/1 -> posedge6/1
  posedge6/1 -> dimm2/1(rst), dimm1/1(rst)
  Counter8/1 -> sync_check2_2/1
  posedge7/1 -> Counter8/1
  sync_check2_2/1 -> Terminator5/1
  Constant1/1 -> Counter1/2
  Constant6/1 -> Counter2/2

== system seti_ct/sys/dram_in ==
  din : Inport  Port=1  LatchInput=off
  sync : Inport  Port=2  LatchInput=off
  Concat : xbsIndex_r3/Concat  num_inputs=2  explicit_period=off  period=1  dbl_ovrd=off
  Counter : xbsIndex_r3/Counter  cnt_type=Free Running  n_bits=2  bin_pt=0  arith_type=Unsigned  start_count=0  cnt_to=Inf  cnt_by_val=1  operation=Up  explicit_period=off  period=1  load_pin=off  rst=on  en=on  dbl_ovrd=off  show_param=off  use_rpm=on  gen_core=off
      settings: xl_area=[0, 0, 0, 0, 0, 0, 0]
  Delay1 : xbsIndex_r3/Delay  latency=1  reg_retiming=off  explicit_period=off  period=1  en=off  accept_only_valid=off  init_zero=on  dbl_ovrd=off  show_param=off
      settings: xl_area=[0, 0, 0, 0, 0, 0, 0]
  Delay2 : xbsIndex_r3/Delay  latency=1  reg_retiming=off  explicit_period=off  period=1  en=off  accept_only_valid=off  init_zero=on  dbl_ovrd=off  show_param=off
      settings: xl_area=[0, 0, 0, 0, 0, 0, 0]
  Delay3 : xbsIndex_r3/Delay  latency=2  reg_retiming=off  explicit_period=off  period=1  en=off  accept_only_valid=off  init_zero=on  dbl_ovrd=off  show_param=off
      settings: xl_area=[0, 0, 0, 0, 0, 0, 0]
  Gateway Out1 : xbsIndex_r3/Gateway Out  output_type=Double  nbits=8  bin_pt=6  arith_type=Boolean  quantization=Truncate  overflow=Wrap  hdl_port=off  timing_constraint=None  locs_specified=off  LOCs={}  needs_fixed_name=off  show_param=off
      settings: xl_area=[0, 0, 0, 0, 0, 0, 0]
  Gateway Out5 : xbsIndex_r3/Gateway Out  output_type=Double  nbits=8  bin_pt=6  arith_type=Boolean  quantization=Truncate  overflow=Wrap  hdl_port=off  timing_constraint=None  locs_specified=off  LOCs={}  needs_fixed_name=off  show_param=off
      settings: xl_area=[0, 0, 0, 0, 0, 0, 0]
  HighBit : xbsIndex_r3/Slice  mode=Upper Bit Location + Width  nbits=1  bit1=0  base1=MSB of Input  bit0=0  base0=LSB of Input  boolean_output=on  explicit_period=off  period=1  dbl_ovrd=off
  LowBit : xbsIndex_r3/Slice  mode=Lower Bit Location + Width  nbits=1  bit1=0  base1=MSB of Input  bit0=0  base0=LSB of Input  boolean_output=on  explicit_period=off  period=1  dbl_ovrd=off
  Mux : xbsIndex_r3/Mux  inputs=2  precision=Full  arith_type="Signed  (2's comp)"  n_bits=8  bin_pt=2  quantization=Truncate  overflow=Wrap  latency=0  explicit_period=off  period=1  en=off  dbl_ovrd=off  show_param=off  mux_type=off  use_rpm=off  gen_core=off
      settings: xl_area=[0, 0, 0, 0, 0, 0, 0]
  Register : xbsIndex_r3/Register  init=0  reg_only_valid=off  explicit_period=off  period=1  rst=off  en=on  out_en=off  dbl_ovrd=off  show_param=off
      settings: xl_area=[0, 0, 0, 0, 0, 0, 0]
  Scope : Scope  NumInputPorts=2
      settings: YMin=-5~-5  YMax=5~5  SaveName=ScopeData8
  dbuf_transpose : Subsystem  AncestorBlock=reorder_library/dbuf_transpose  mask{Rows=spec_len, Cols=2, bram_latency=2}
      mask prompts: Rows "Rows of Matrix (data written in): (2^?)"; Cols "Cols of Matrix (data read out): (2^?)"; bram_latency "BRAM Latency"
  is2 : xbsIndex_r3/Expression  expression=~a & b  precision=Full  arith_type=Unsigned  n_bits=8  bin_pt=2  align_bp=on  latency=0  explicit_period=off  period=1  en=off  dbl_ovrd=off  show_param=off
      settings: xl_area=[0, 0, 0, 0, 0, 0, 0]
  dout : Outport
  r_valid : Outport  Port=2
  w_valid : Outport  Port=3
  sync_out : Outport  Port=4
  wires:
  dbuf_transpose/2(sync_out) -> Counter/1, Register/1, Delay3/1, Register/2, Gateway Out1/1
  Delay1/1 -> Concat/2
  dbuf_transpose/1(dout) -> Delay1/1, Concat/1, Gateway Out5/1
  sync/1 -> dbuf_transpose/2(sync)
  din/1 -> dbuf_transpose/1(din)
  Counter/1 -> HighBit/1, LowBit/1
  Mux/1 -> dout/1
  Concat/1 -> Mux/3, Delay2/1
  Delay2/1 -> Mux/2
  LowBit/1 -> Mux/1, is2/1
  Delay3/1 -> sync_out/1
  is2/1 -> r_valid/1
  HighBit/1 -> is2/2, w_valid/1
  Register/1 -> Counter/2
  Gateway Out5/1 -> Scope/1
  Gateway Out1/1 -> Scope/2

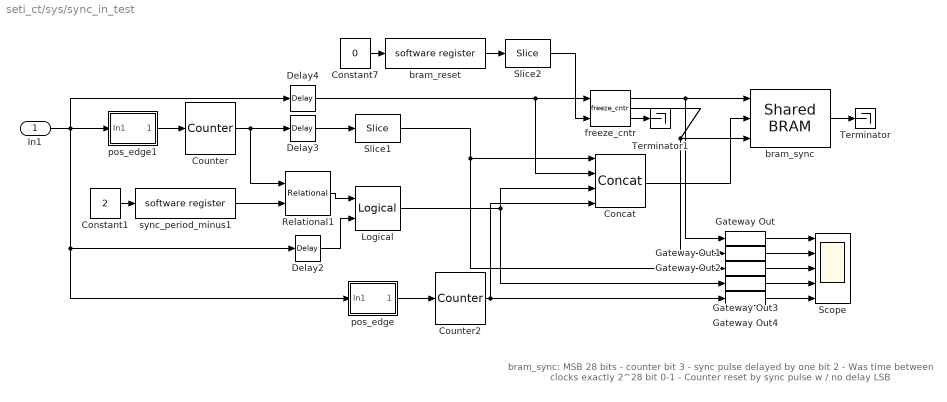
== system seti_ct/sys/sync_in_test ==
  note: bram_sync: MSB
      | 28 bits - counter
      | bit 3 - sync pulse delayed by one
      | bit 2 - Was time between clocks exactly 2^28
      | bit 0-1 - Counter reset by sync pulse w / no delay
      | LSB
  In1 : Inport  Port=1  LatchInput=off
  Concat : xbsIndex_r3/Concat  num_inputs=4  explicit_period=off  period=1  dbl_ovrd=off
  Constant1 : Constant  Value=2
  Constant7 : Constant  Value=0
  Counter : xbsIndex_r3/Counter  cnt_type=Free Running  n_bits=32  bin_pt=0  arith_type=Unsigned  start_count=0  cnt_to=2^4-1  cnt_by_val=1  operation=Up  explicit_period=on  period=1  load_pin=off  rst=on  en=off  dbl_ovrd=off  show_param=off  use_rpm=on  gen_core=off
      settings: xl_area=[0, 0, 0, 0, 0, 0, 0]
  Counter2 : xbsIndex_r3/Counter  cnt_type=Count Limited  n_bits=2  bin_pt=0  arith_type=Unsigned  start_count=0  cnt_to=3  cnt_by_val=1  operation=Up  explicit_period=on  period=1  load_pin=off  rst=on  en=off  dbl_ovrd=off  show_param=off  use_rpm=on  gen_core=off
      settings: xl_area=[0, 0, 0, 0, 0, 0, 0]
  Delay2 : xbsIndex_r3/Delay  latency=1  reg_retiming=off  explicit_period=on  period=1  en=off  accept_only_valid=off  init_zero=on  dbl_ovrd=off  show_param=off
      settings: xl_area=[0, 0, 0, 0, 0, 0, 0]
  Delay3 : xbsIndex_r3/Delay  latency=1  reg_retiming=off  explicit_period=on  period=1  en=off  accept_only_valid=off  init_zero=on  dbl_ovrd=off  show_param=off
      settings: xl_area=[0, 0, 0, 0, 0, 0, 0]
  Delay4 : xbsIndex_r3/Delay  latency=1  reg_retiming=off  explicit_period=on  period=1  en=off  accept_only_valid=off  init_zero=on  dbl_ovrd=off  show_param=off
      settings: xl_area=[0, 0, 0, 0, 0, 0, 0]
  Gateway Out{,1..4} (5 alike) : xbsIndex_r3/Gateway Out  output_type=Double  nbits=8  bin_pt=6  arith_type=Boolean  quantization=Truncate  overflow=Wrap  hdl_port=on  timing_constraint=None  locs_specified=off  LOCs={}  needs_fixed_name=off  show_param=off
      settings: xl_area=[0, 0, 0, 0, 0, 0, 0]
  Logical : xbsIndex_r3/Logical  logical_function=AND  inputs=2  precision=Full  arith_type=Unsigned  n_bits=2  bin_pt=0  align_bp=on  latency=0  explicit_period=off  period=1  en=off  dbl_ovrd=off  show_param=off
      settings: xl_area=[0, 0, 0, 0, 0, 0, 0]
  Relational1 : xbsIndex_r3/Relational  mode=a=b  latency=1  explicit_period=on  period=1  en=off  dbl_ovrd=off  show_param=off
      settings: xl_area=[0, 0, 0, 0, 0, 0, 0]
  Scope : Scope  NumInputPorts=5
      settings: YMin=-5~-5~-5~-5~-5  YMax=5~5~5~5~5
  Slice1 : xbsIndex_r3/Slice  mode=Lower Bit Location + Width  nbits=28  bit1=0  base1=MSB of Input  bit0=0  base0=LSB of Input  boolean_output=off  explicit_period=off  period=1  dbl_ovrd=off
  Slice2 : xbsIndex_r3/Slice  mode=Lower Bit Location + Width  nbits=1  bit1=0  base1=MSB of Input  bit0=0  base0=LSB of Input  boolean_output=on  explicit_period=off  period=1  dbl_ovrd=off
  Terminator : Terminator
  Terminator1 : Terminator
  bram_reset : xps_library/software register  Tag=xps:sw_reg  io_dir=From Processor  arith_type=Unsigned  bitwidth=32  bin_pt=0  sample_period=1  gw_name=seti_ct_sys_sync_in_test_bram_reset_user_data_out
  bram_sync : xps_library/Shared BRAM  Tag=xps:bram  arith_type=Unsigned  addr_width=12  data_width=32  data_bin_pt=0  init_vals=0  sample_rate=1
  freeze_cntr : casper_library/Misc/freeze_cntr  CounterBits=12
  pos_edge : Subsystem
  pos_edge1 : Subsystem
  sync_period_minus1 : xps_library/software register  Tag=xps:sw_reg  io_dir=From Processor  arith_type=Unsigned  bitwidth=32  bin_pt=0  sample_period=1  gw_name=seti_ct_sys_sync_in_test_sync_period_minus1_user_data_out
  wires:
  Counter/1 -> Relational1/1, Delay3/1
  Relational1/1 -> Logical/1
  Delay2/1 -> Logical/2
  Constant1/1 -> sync_period_minus1/1
  sync_period_minus1/1 -> Relational1/2
  freeze_cntr/1 -> bram_sync/1, Gateway Out/1
  freeze_cntr/2 -> bram_sync/3, Gateway Out1/1
  Delay3/1 -> Slice1/1
  Delay4/1 -> Concat/2, freeze_cntr/1
  Constant7/1 -> bram_reset/1
  bram_reset/1 -> Slice2/1
  Gateway Out/1 -> Scope/1
  Gateway Out1/1 -> Scope/2
  Gateway Out2/1 -> Scope/3
  Gateway Out3/1 -> Scope/4
  Concat/1 -> bram_sync/2
  Logical/1 -> Gateway Out3/1, Concat/3
  Slice2/1 -> freeze_cntr/2
  Gateway Out4/1 -> Scope/5
  pos_edge/1(Out1) -> Counter2/1
  Counter2/1 -> Gateway Out4/1, Concat/4
  pos_edge1/1(Out1) -> Counter/1
  Slice1/1 -> Concat/1, Gateway Out2/1
  In1/1 -> pos_edge1/1(In1), Delay4/1, Delay2/1, pos_edge/1(In1)
  bram_sync/1 -> Terminator/1
  freeze_cntr/3 -> Terminator1/1
